simulink model "TemplateMatchingContinuous"  (R2020a)
settings: Solver=VariableStepAuto  StartTime=0.0  StopTime=40  RelTol=1e-3
libraries: simulink x2, dspswit3 x1, dspfdesign x1, hdlsllib x1
settings Model: Creator=sbuccelli  LastModifiedBy=diflo

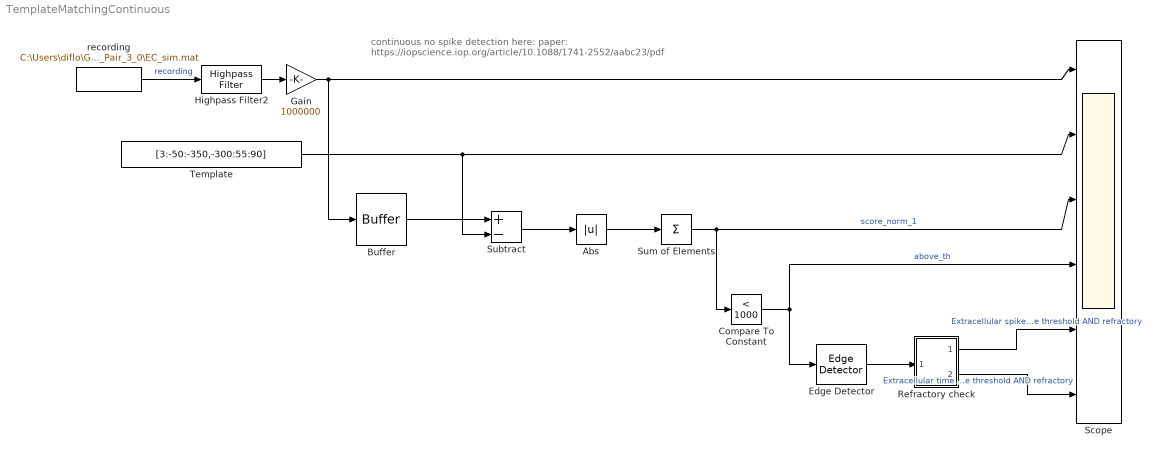
== system TemplateMatchingContinuous ==
  note: continuous no spike detection here:
      | paper: https://iopscience.iop.org/article/10.1088/1741-2552/aabc23/pdf
  Abs : Abs
  Buffer : Buffer  N=16  V=15  OutputFrames=off
  Compare To Constant : simulink/Logic and Bit Operations/Compare To Constant  relop=<  const=1000  OutDataTypeStr=boolean
  Edge Detector : dspswit3/Edge Detector  InputProcessing=Columns as channels (frame based)
      settings: SourceProductBaseCode=DS
  Gain : Gain  Gain=1000000
  Highpass Filter2 : dspfdesign/Highpass Filter  FilterType=IIR  DesignForMinimumOrder=off  FilterOrder=3  StopbandFrequency=1  PassbandFrequency=300  StopbandAttenuation=80  PassbandRipple=0.1  InheritSampleRate=off  SampleRate=30000  SimulateUsing=Interpreted execution  roundingMode=Floor  coeffsDataTypeStr=fixdt(1,16)
  Refractory check : Subsystem
  Scope : Scope  NumInputPorts=6
  Subtract : Sum  Inputs=+-
  Sum of Elements : Sum  Inputs=+
  Template : Constant  Value=[3:-50:-350,-300:55:90]  SampleTime=1/30000
  recording : FromFile  FileName=C:\Users\diflo\Google Drive\IIT - Neuroengineering\MathWorks Project\Data\KampffLab\2014_11_25_Pair_3_0\EC_sim.mat  SampleTime=1/30000
  wires:
  recording/1 -> Highpass Filter2/1  "recording"
  Buffer/1 -> Subtract/1
  Subtract/1 -> Abs/1
  Abs/1 -> Sum of Elements/1
  Sum of Elements/1 -> Compare To Constant/1, Scope/3  "score_norm_1"
  Template/1 -> Subtract/2, Scope/2
  Compare To Constant/1 -> Scope/4, Edge Detector/1  "above_th"
  Gain/1 -> Buffer/1, Scope/1
  Highpass Filter2/1 -> Gain/1
  Edge Detector/1 -> Refractory check/1("   ")
  Refractory check/1(" ") -> Scope/5  "Extracellular spikes above threshold AND refractory"
  Refractory check/2(Output) -> Scope/6  "Extracellular time since last spike above threshold AND refractory"

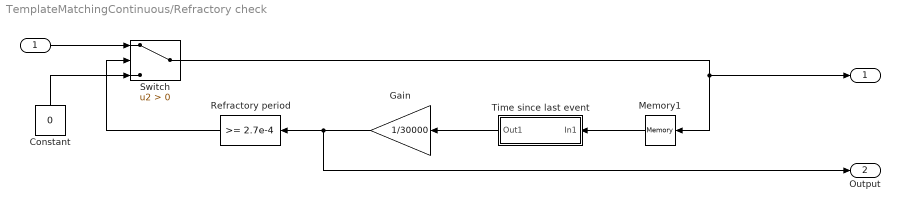
== system TemplateMatchingContinuous/Refractory check ==
  "   " : Inport
  Constant : Constant  Value=0
  Gain : Gain  Gain=1/30000  ParamDataTypeStr=double
  Memory1 : Memory  InheritSampleTime=on
  Refractory period : simulink/Logic and Bit Operations/Compare To Constant  relop=>=  const=2.7e-4  OutDataTypeStr=boolean
  Switch : Switch  Criteria=u2 > Threshold
  Time since last event : Subsystem
  " " : Outport
  Output : Outport  Port=2
  wires:
  "   "/1 -> Switch/1
  Memory1/1 -> Time since last event/1(In1)
  Time since last event/1(Out1) -> Gain/1
  Constant/1 -> Switch/3
  Gain/1 -> Refractory period/1, Output/1
  Switch/1 -> " "/1, Memory1/1
  Refractory period/1 -> Switch/2

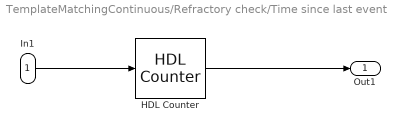
== system TemplateMatchingContinuous/Refractory check/Time since last event ==
  In1 : Inport
  HDL Counter : hdlsllib/Sources/HDL Counter  CountType=Free running  CountInit=1  CountStep=1  CountMax=25  CountFromType=Initial value  CountFrom=1  CountResetPort=on  CountLoadPort=off  CountEnbPort=off  CountDirPort=off  CountDataType=Unsigned  CountWordLen=32  CountFracLen=0  CountSampTime=1
  Out1 : Outport
  wires:
  In1/1 -> HDL Counter/1
  HDL Counter/1 -> Out1/1
